simulink model "lab_ready"  (R2020b)
settings: Solver=ode4  StartTime=0.0  StopTime=50  FixedStep=0.001  RelTol=1e-3
values from neighbouring files (symbols this model uses):
  degs2rpm = 0.166666666667    [DIGIT1-BE10.mat]    (also in DIGIT1-FE10.mat; DIGIT1-FE20.mat; DIGIT1-FE4.mat; DIGIT1-TR10.mat)
  filt =     [DIGIT1-BE10.mat]    (also in DIGIT1-FE10.mat; DIGIT1-FE20.mat; DIGIT1-FE4.mat; DIGIT1-TR10.mat)
  rpm2rads = 0.10471975512    [DIGIT1-BE10.mat]    (also in DIGIT1-FE10.mat; DIGIT1-FE20.mat; DIGIT1-FE4.mat; DIGIT1-TR10.mat)
undefined symbols (not defined in the file or in its folder): National_Instruments, PCI
libraries: sldrtlib x3, simulink x3
settings Model: ExtModeTrigDuration=50001  Creator=verrimarco  LastModifiedBy=verrimarco
settings DataIOCC: SaveFormat=StructureWithTime  ReturnWorkspaceOutputs=off  LoggingFileName=out.mat2
settings RTWCC: Description=Simulink Desktop Real-Time  SystemTargetFile=sldrt.tlc  TemplateMakefile=sldrt.tmf  RTWCompilerOptimization=on
settings CodeAppCC: MaxIdLength=95
settings SimulinkDesktopRealTimeCC: TargetPreCompLibLocation=C:\Program Files\MATLAB\R2020b\toolbox\sldrt\lib\win64

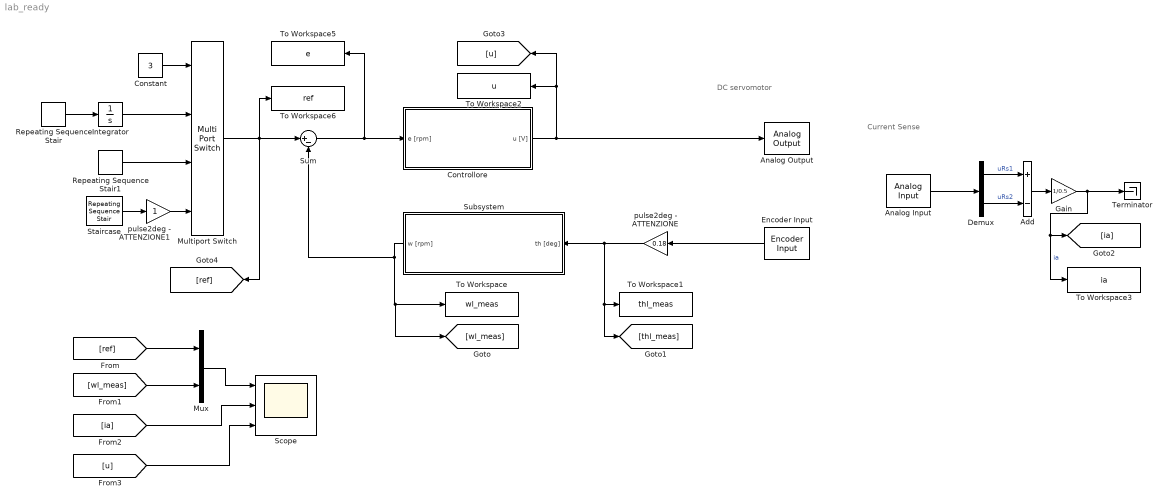
== system lab_ready ==
  note: DC servomotor
  note: Current Sense
  Add : Sum  Inputs=+-
  Analog Input : sldrtlib/Analog Input  SampleTime=-1  MaxMissedTicks=10  ShowMissedTicks=off  YieldWhenWaiting=off  DrvName=National_Instruments/PCI-6221  DrvAddress=4294967295  DrvOptions=[0 0 0 2 0]  Channels=[1,2]  RangeMode=1  VoltRange=1  DataType=1
      settings: AttributesFormatString=National Instruments\nPCI-6221 [auto]
  Analog Output : sldrtlib/Analog Output  SampleTime=-1  MaxMissedTicks=10  ShowMissedTicks=off  YieldWhenWaiting=off  DrvName=National_Instruments/PCI-6221  DrvAddress=4294967295  DrvOptions=[0 0 0 2 0]  Channels=1  RangeMode=1  VoltRange=1  InitialValue=0  FinalValue=0
      settings: AttributesFormatString=National Instruments\nPCI-6221 [auto]
  Constant : Constant  Value=3
  Controllore : Subsystem
  Demux : Demux  Outputs=2
  Encoder Input : sldrtlib/Encoder Input  SampleTime=-1  MaxMissedTicks=10  ShowMissedTicks=off  YieldWhenWaiting=on  DrvName=National_Instruments/PCI-6221  DrvAddress=4294967295  DrvOptions=[0 0 0 2 0]  Channels=1  QuadMode=3  IndexPulse=1  InputFilter=Inf  DataType=1
      settings: AttributesFormatString=National Instruments\nPCI-6221 [auto]
  Gain : Gain  Gain=1/0.5
  Integrator : Integrator
  Multiport Switch : MultiPortSwitch
  Mux : Mux  Inputs=2
  Repeating Sequence Stair : simulink/Sources/Repeating Sequence Stair  OutValues=[450 -450].'  tsamp=1  OutMin=[]  OutMax=[]  OutDataTypeStr=double  OutputDataTypeScalingMode=double  OutDataType=fixdt(0,8)  ConRadixGroup=Best Precision: Vector-wise  OutScaling=2^-12
  Repeating Sequence Stair1 : simulink/Sources/Repeating Sequence Stair  OutValues=[250 -250].'  tsamp=1.5  OutMin=[]  OutMax=[]  OutDataTypeStr=double  OutputDataTypeScalingMode=double  OutDataType=fixdt(0,8)  ConRadixGroup=Best Precision: Vector-wise  OutScaling=2^-12
  Scope : Scope  NumInputPorts=3
  Staircase : simulink/Sources/Repeating Sequence Stair  OutValues=[0 50 100 150 200 250 300 350 400 450 450].'  tsamp=5  OutMin=[]  OutMax=[]  OutDataTypeStr=double  OutputDataTypeScalingMode=double  OutDataType=fixdt(0,8)  ConRadixGroup=Best Precision: Vector-wise  OutScaling=2^-12
  Subsystem : Subsystem
  Sum : Sum  Inputs=|+-
  Terminator : Terminator
  To Workspace : ToWorkspace  VariableName=wl_meas  SaveFormat=Structure With Time  SampleTime=-1
  To Workspace1 : ToWorkspace  VariableName=thl_meas  SaveFormat=Structure With Time  SampleTime=-1
  To Workspace2 : ToWorkspace  VariableName=u  SaveFormat=Structure With Time  SampleTime=-1
  To Workspace3 : ToWorkspace  VariableName=ia  SaveFormat=Structure With Time  SampleTime=-1
  To Workspace5 : ToWorkspace  VariableName=e  SaveFormat=Structure With Time  SampleTime=-1
  To Workspace6 : ToWorkspace  VariableName=ref  SaveFormat=Structure With Time  SampleTime=-1
  pulse2deg - ATTENZIONE : Gain  Gain=0.18
  pulse2deg - ATTENZIONE1 : Gain
  wires:
  Analog Input/1 -> Demux/1
  Demux/1 -> Add/1  "uRs1"
  Demux/2 -> Add/2  "uRs2"
  Add/1 -> Gain/1
  Gain/1 -> To Workspace3/1, [ia], Terminator/1  "ia"
  Controllore/1(u [V]) -> To Workspace2/1, [u], Analog Output/1
  pulse2deg - ATTENZIONE/1 -> [thl_meas], To Workspace1/1, Subsystem/1(th [deg])
  Encoder Input/1 -> pulse2deg - ATTENZIONE/1
  Subsystem/1(w [rpm]) -> Sum/2, [wl_meas], To Workspace/1
  Repeating Sequence Stair/1 -> Integrator/1
  Sum/1 -> To Workspace5/1, Controllore/1(e [rpm])
  Constant/1 -> Multiport Switch/1
  Repeating Sequence Stair1/1 -> Multiport Switch/3
  Integrator/1 -> Multiport Switch/2
  Multiport Switch/1 -> [ref], To Workspace6/1, Sum/1
  [wl_meas] -> Mux/2
  [ref] -> Mux/1
  Mux/1 -> Scope/1
  [ia] -> Scope/2
  [u] -> Scope/3
  pulse2deg - ATTENZIONE1/1 -> Multiport Switch/4
  Staircase/1 -> pulse2deg - ATTENZIONE1/1

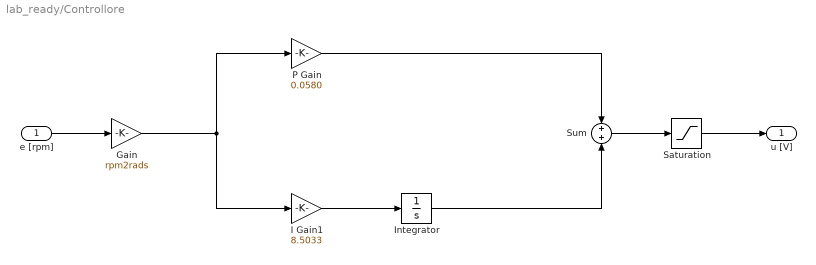
== system lab_ready/Controllore ==
  e [rpm] : Inport
  Gain : Gain  Gain=rpm2rads
  I Gain1 : Gain  Gain=8.5033
  Integrator : Integrator
  P Gain : Gain  Gain=0.0580
  Saturation : Saturate  UpperLimit=12  LowerLimit=-12
  Sum : Sum
  u [V] : Outport
  wires:
  e [rpm]/1 -> Gain/1
  I Gain1/1 -> Integrator/1
  Integrator/1 -> Sum/2
  P Gain/1 -> Sum/1
  Gain/1 -> I Gain1/1, P Gain/1
  Saturation/1 -> u [V]/1
  Sum/1 -> Saturation/1

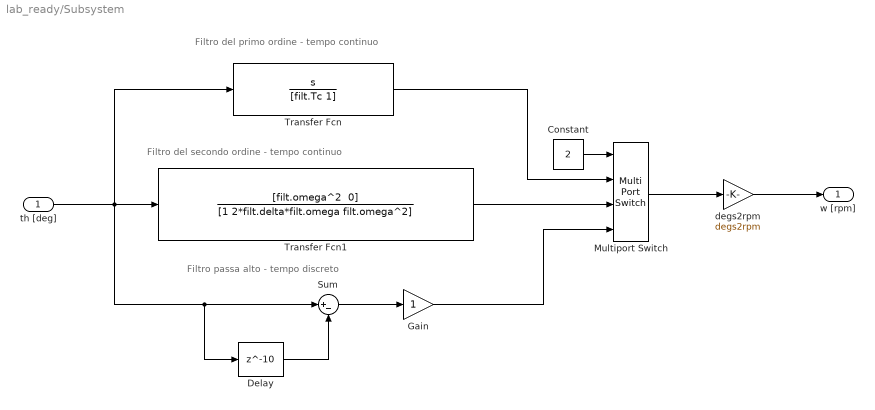
== system lab_ready/Subsystem ==
  note: Filtro passa alto - tempo discreto
  note: Filtro del secondo ordine - tempo continuo
  note: Filtro del primo ordine - tempo continuo
  th [deg] : Inport
  Constant : Constant  Value=2
  Delay : Delay  DelayLength=10  InitialCondition=0
  Gain : Gain
  Multiport Switch : MultiPortSwitch
  Sum : Sum  Inputs=|+-
  Transfer Fcn : TransferFcn  Numerator=[1 0]  Denominator=[filt.Tc 1]
  Transfer Fcn1 : TransferFcn  Numerator="[filt.omega^2  0]"  Denominator=[1 2*filt.delta*filt.omega filt.omega^2]
  degs2rpm : Gain  Gain=degs2rpm
  w [rpm] : Outport
  wires:
  Delay/1 -> Sum/2
  Sum/1 -> Gain/1
  th [deg]/1 -> Delay/1, Sum/1, Transfer Fcn1/1, Transfer Fcn/1
  Transfer Fcn1/1 -> Multiport Switch/3
  Transfer Fcn/1 -> Multiport Switch/2
  Gain/1 -> Multiport Switch/4
  Constant/1 -> Multiport Switch/1
  Multiport Switch/1 -> degs2rpm/1
  degs2rpm/1 -> w [rpm]/1
